simulink model "xeng_tvg_test"  (Simulink 7.0)
settings: Solver=VariableStepDiscrete  StartTime=0.0  StopTime=1200  RelTol=1e-3
libraries: xbsIndex_r4 x24, casper_library x5, simulink x3
settings Model: Creator=User  LastModifiedBy=User
settings DebuggingCC: SaveWithDisabledLinksMsg=none  SaveWithParameterizedLinksMsg=none

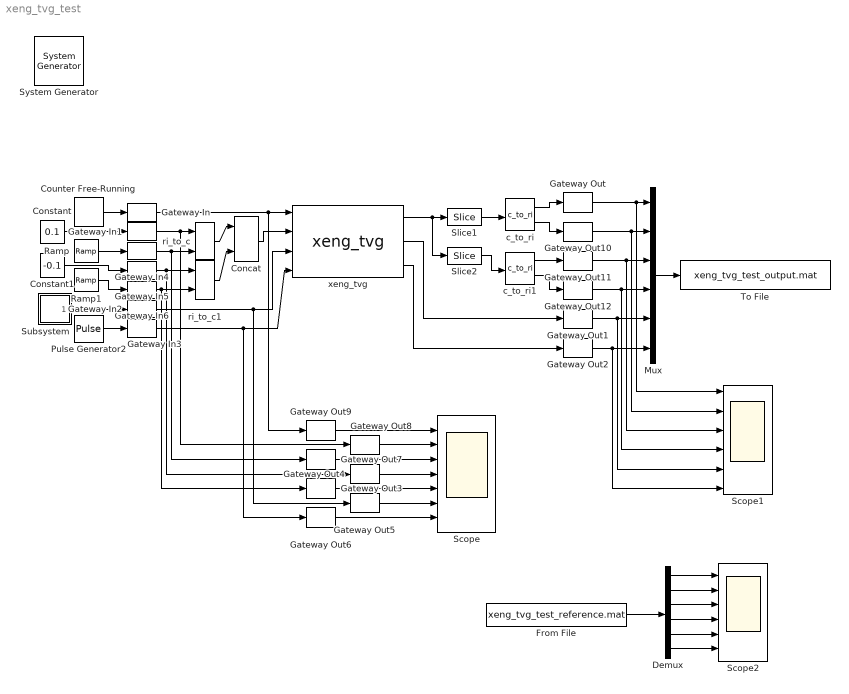
== system xeng_tvg_test ==
  " System Generator" : xbsIndex_r4/ System Generator  Tag=genX  SystemSampleTime=-1  xilinxfamily=Virtex4  part=xc4vsx35  speed=-10  package=ff668  synthesis_tool=XST  clock_wrapper=Clock Enables  directory=./netlist  testbench=off  simulink_period=1  sysclk_period=100  dcm_input_clock_period=100  incr_netlist=off  trim_vbits=Everywhere in SubSystem  dbl_ovrd=According to Block Masks  core_generation=According to Block Masks  run_coregen=off  deprecated_control=off  eval_field=0  block_type=sysgen
      settings: block_version=10.1.1
  Concat : xbsIndex_r4/Concat  num_inputs=2  dbl_ovrd=off  block_type=concat
      settings: block_version=10.1.1
  Constant : Constant  Value=0.1  OutDataType=sfix(16)  OutScaling=2^0
  Constant1 : Constant  Value=-0.1  OutDataType=sfix(16)  OutScaling=2^0
  Counter Free-Running : simulink/Sources/Counter Free-Running  SystemSampleTime=-1  NumBits=2  tsamp=2^(4+4)
  Demux : Demux  Outputs=6
  From File : FromFile  FileName=xeng_tvg_test_reference.mat  SampleTime=0
  Gateway In : xbsIndex_r4/Gateway In  arith_type=Unsigned  n_bits=2  bin_pt=0  quantization=Truncate  overflow=Wrap  period=1  dbl_ovrd=off  timing_constraint=None  locs_specified=off  LOCs={}  block_type=gatewayin
      settings: infoedit="Gateway in block.  Converts inputs of type Simulink integer, double and fixed point to  Xilinx fixed point type.<P><P>Hardware notes:  In hardware these blocks become top level input ports."  block_version=10.1.1
  Gateway In{1,4..6} (4 alike) : xbsIndex_r4/Gateway In  arith_type="Signed  (2's comp)"  n_bits=8  bin_pt=7  quantization=Truncate  overflow=Wrap  period=1  dbl_ovrd=off  timing_constraint=None  locs_specified=off  LOCs={}  block_type=gatewayin
      settings: infoedit="Gateway in block.  Converts inputs of type Simulink integer, double and fixed point to  Xilinx fixed point type.<P><P>Hardware notes:  In hardware these blocks become top level input ports."  block_version=10.1.1
  Gateway In2 : xbsIndex_r4/Gateway In  arith_type=Boolean  n_bits=8  bin_pt=0  quantization=Truncate  overflow=Wrap  period=1  dbl_ovrd=off  timing_constraint=None  locs_specified=off  LOCs={}  block_type=gatewayin
      settings: infoedit="Gateway in block.  Converts inputs of type Simulink integer, double and fixed point to  Xilinx fixed point type.<P><P>Hardware notes:  In hardware these blocks become top level input ports."  block_version=10.1.1
  Gateway In3 : xbsIndex_r4/Gateway In  arith_type=Boolean  n_bits=8  bin_pt=0  quantization=Truncate  overflow=Wrap  period=1  dbl_ovrd=off  timing_constraint=None  locs_specified=off  LOCs={}  block_type=gatewayin
      settings: infoedit="Gateway in block.  Converts inputs of type Simulink integer, double and fixed point to  Xilinx fixed point type.<P><P>Hardware notes:  In hardware these blocks become top level input ports."  block_version=10.1.1
  Gateway Out{,1..12} (13 alike) : xbsIndex_r4/Gateway Out  hdl_port=on  timing_constraint=None  locs_specified=off  LOCs={}  block_type=gatewayout
      settings: infoedit="Gateway out block.  Converts Xilinx fixed point inputs into ouputs of type Simulink integer, double, or fixed point.<P><P>Hardware notes:  In hardware these blocks become top level output ports or are discarded, depending on how they are configured."  block_version=10.1.1
  Mux : Mux  Inputs=6
  Pulse Generator2 : DiscretePulseGenerator  Period=2^9  PhaseDelay=7
  Ramp : simulink/Sources/Ramp  SystemSampleTime=-1  slope=1/2^8  start=0  X0=0
  Ramp1 : simulink/Sources/Ramp  SystemSampleTime=-1  slope=1/2^6  start=0  X0=0
  Scope : Scope  NumInputPorts=7
      settings: YMin=-5~-5~-5~-5~-5~-5~-5  YMax=5~5~5~5~5~5~5
  Scope1 : Scope  NumInputPorts=6
      settings: YMin=-1~-5~-5~-5~-5~-5  YMax=1~5~5~5~5~5
  Scope2 : Scope  NumInputPorts=6
      settings: YMin=-5~-5~-5~-5~-5~-5  YMax=5~5~5~5~5~5  SaveName=ScopeData2
  Slice1 : xbsIndex_r4/Slice  nbits=16  boolean_output=off  mode=Upper Bit Location + Width  bit1=0  base1=MSB of Input  bit0=0  base0=LSB of Input  dbl_ovrd=off  block_type=slice
      settings: infoedit="Extracts a given range of bits from each input sample and presents it at the output.  The output type is ordinarily unsigned with binary point at zero, but can be Boolean when the slice is one bit wide.<P><P>Hardware notes: In hardware this block costs nothing."  block_version=10.1.1
  Slice2 : xbsIndex_r4/Slice  nbits=16  boolean_output=off  mode=Lower Bit Location + Width  bit1=0  base1=MSB of Input  bit0=0  base0=LSB of Input  dbl_ovrd=off  block_type=slice
      settings: infoedit="Extracts a given range of bits from each input sample and presents it at the output.  The output type is ordinarily unsigned with binary point at zero, but can be Boolean when the slice is one bit wide.<P><P>Hardware notes: In hardware this block costs nothing."  block_version=10.1.1
  Subsystem : Subsystem
  To File : ToFile  Filename=xeng_tvg_test_output.mat  MatrixName=output
  c_to_ri : casper_library/Misc/c_to_ri  SystemSampleTime=-1  n_bits=8  bin_pt=7
      settings: AttributesFormatString=8_7 r/i
  c_to_ri1 : casper_library/Misc/c_to_ri  SystemSampleTime=-1  n_bits=8  bin_pt=7
      settings: AttributesFormatString=8_7 r/i
  ri_to_c : casper_library/Misc/ri_to_c  SystemSampleTime=-1
  ri_to_c1 : casper_library/Misc/ri_to_c  SystemSampleTime=-1
  xeng_tvg : casper_library/Correlator/xeng_tvg  SystemSampleTime=-1  ant_bits=4  bits_in=8  x_int_bits=4  sync_period=9
      link override tv0/xeng_tvg_test_xeng_tvg_tv0_user_data_out: arith_type=Unsigned  n_bits=32  bin_pt=0  period=1
      link override tv1/xeng_tvg_test_xeng_tvg_tv1_user_data_out: arith_type=Unsigned  n_bits=32  bin_pt=0  period=1
      link override tv2/xeng_tvg_test_xeng_tvg_tv2_user_data_out: arith_type=Unsigned  n_bits=32  bin_pt=0  period=1
      link override tv3/xeng_tvg_test_xeng_tvg_tv3_user_data_out: arith_type=Unsigned  n_bits=32  bin_pt=0  period=1
      link override tv4/xeng_tvg_test_xeng_tvg_tv4_user_data_out: arith_type=Unsigned  n_bits=32  bin_pt=0  period=1
      link override tv5/xeng_tvg_test_xeng_tvg_tv5_user_data_out: arith_type=Unsigned  n_bits=32  bin_pt=0  period=1
      link override tv6/xeng_tvg_test_xeng_tvg_tv6_user_data_out: arith_type=Unsigned  n_bits=32  bin_pt=0  period=1
      link override tv7/xeng_tvg_test_xeng_tvg_tv7_user_data_out: arith_type=Unsigned  n_bits=32  bin_pt=0  period=1
  wires:
  Counter Free-Running/1 -> Gateway In/1
  Gateway In/1 -> xeng_tvg/1, Gateway Out9/1
  Subsystem/1(Out1) -> Gateway In2/1
  Gateway In2/1 -> xeng_tvg/3, Gateway Out5/1
  Pulse Generator2/1 -> Gateway In3/1
  Gateway In3/1 -> xeng_tvg/4, Gateway Out6/1
  xeng_tvg/2 -> Gateway Out1/1
  xeng_tvg/3 -> Gateway Out2/1
  Mux/1 -> To File/1
  Constant/1 -> Gateway In1/1
  Ramp/1 -> Gateway In4/1
  Constant1/1 -> Gateway In5/1
  Ramp1/1 -> Gateway In6/1
  Gateway In1/1 -> Gateway Out8/1, ri_to_c/1
  Gateway In4/1 -> Gateway Out7/1, ri_to_c/2
  Gateway In5/1 -> ri_to_c1/1, Gateway Out4/1
  Gateway In6/1 -> ri_to_c1/2, Gateway Out3/1
  ri_to_c/1 -> Concat/1
  ri_to_c1/1 -> Concat/2
  Concat/1 -> xeng_tvg/2
  Gateway Out9/1 -> Scope/1
  Gateway Out8/1 -> Scope/2
  Gateway Out7/1 -> Scope/3
  Gateway Out4/1 -> Scope/4
  Gateway Out3/1 -> Scope/5
  Gateway Out5/1 -> Scope/6
  Gateway Out6/1 -> Scope/7
  xeng_tvg/1 -> Slice1/1, Slice2/1
  Slice1/1 -> c_to_ri/1
  Slice2/1 -> c_to_ri1/1
  c_to_ri/1 -> Gateway Out/1
  c_to_ri/2 -> Gateway Out10/1
  c_to_ri1/1 -> Gateway Out11/1
  c_to_ri1/2 -> Gateway Out12/1
  Gateway Out/1 -> Mux/1, Scope1/1
  Gateway Out10/1 -> Mux/2, Scope1/2
  Gateway Out11/1 -> Mux/3, Scope1/3
  Gateway Out12/1 -> Mux/4, Scope1/4
  Gateway Out1/1 -> Mux/5, Scope1/5
  Gateway Out2/1 -> Mux/6, Scope1/6
  From File/1 -> Demux/1
  Demux/1 -> Scope2/1
  Demux/2 -> Scope2/2
  Demux/3 -> Scope2/3
  Demux/4 -> Scope2/4
  Demux/5 -> Scope2/5
  Demux/6 -> Scope2/6

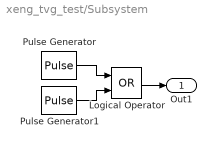
== system xeng_tvg_test/Subsystem ==
  Logical Operator : Logic  Operator=OR  AllPortsSameDT=off  OutDataTypeMode=boolean
  Pulse Generator : DiscretePulseGenerator  Period=2^4  PulseWidth=2^4-1  PhaseDelay=3
  Pulse Generator1 : DiscretePulseGenerator  Period=2^5  PulseWidth=2^5-1  PhaseDelay=3
  Out1 : Outport
  wires:
  Pulse Generator/1 -> Logical Operator/1
  Pulse Generator1/1 -> Logical Operator/2
  Logical Operator/1 -> Out1/1
